simulink library "wtd_library_ver1"  (R2014b)
settings: Solver=ode45  StartTime=0.0  StopTime=10.0  RelTol=1e-3
undefined symbols (not defined in the file or in its folder): clearaugYMatrix, complexPower, dwo, faultaugYMatrix, genTranReactance, invclearaugYMatrix, invfaultaugYMatrix, invsystemaugYMatrix, j, nodeVoltage, noGridNodes, pffault_set_global, s3cc, tho
undefined symbols (not defined in the file): baseSystemPower, internalGenVoltage, pitchAngleVec, systemFrequency, turbSpeedVec, windturbKaParam, windturbKbParam, WTD_Y12, WTD_Y12_2
libraries: simulink x18
(part 1 of 3)
settings Model: Creator=Jakub  LastModifiedBy=Jakub

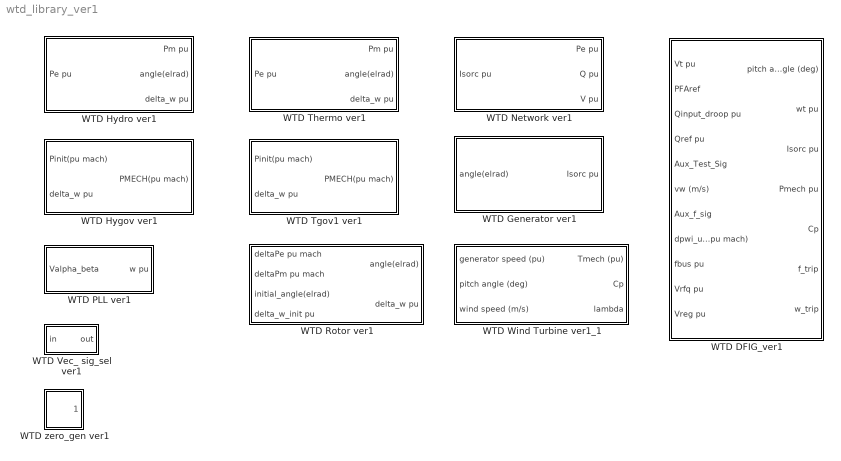
== system wtd_library_ver1 ==
  WTD DFIG_ver1 : Subsystem  mask{co_node=4, Sbasesys=baseSystemPower, Sbasem4=100.5, wbase=2*pi*systemFrequency, H=4.94, Xsecsys=genTranReactance, Ka=windturbKaParam, Kb=windturbKbParam, Vwinit=nodeVoltage, Pelec4abs=real(complexPower)*baseSystemPower, Qgen4abs=imag(complexPower)*baseSystemPower, theta=pitchAngleVec, w=turbSpeedVec, pfaflg=0, varflg=1, apcflg=0, Kqd=0, Kpv=18, Kiv=5, Qmax=0.436, Qmin=-0.436, KVi=40, insupp=0, wi_user_GE=0, Kwi=10, Kptrq=3, Kitrq=0.6, Tpc=0.05, dbwi=0.0025, TIpwi=1, Twowi=5.5, urlwi=0.1, drlwi=-1, Pmxwi=0.1, Pmnwi=0}
      mask prompts: co_node "Connection node number"; Sbasesys "Base system power (MVA)"; Sbasem4 "Nominal machine power (MVA)"; wbase "Base system speed"; H "Machine inertial constant H (s)"; Xsecsys "xdprim (pu sys)"; Vwinit "Initial bus voltage (pu real+j*imag)"; Pelec4abs "Initial active power (MW)"; Qgen4abs "Initial reactive power (MVAr)"; theta "Inital pitch angle (rad)"; w "Inital wind turbine speed (pu)"; pfaflg "Power factor regulation or Q regulation (pfaflg)"; varflg "Voltage regulation, PFA or Q, Q sep. mod. (varflg)"; apcflg "Active power control enabled (apcflg)"; Kqd "Q droop gain Kqd"; Kpv "Reactive power control Kpv"; Kiv "Reactive power control Kiv"; Qmax "Reactive power control qmax"; Qmin "Reactive power control qmin"; KVi "Electrical control Kvi"; insupp "Inertial support (yes = 1, no = 0)"; wi_user_GE "Inertial support: Ge - 0 or User - 1"
      mask init:
      | %DFIG state initialization 
      | %%Generator Converter Model GE
      |     Tcon=0.02;     %converter time constant (s)
      |     %LVPL (low voltage power logic)
      |     zerox=0.2; %0.5  
      |     brkpt=0.9;
      |     LVPLhigh=1.22;
      |     LVPLlow=0;
      |     rrpwr=10;
      |     %Low voltage active current management
      |     lvpnt0=0;%0.4 %Low voltage active current management breakpoint (pu)
      |     lvpnt1=0.8; %Low voltage active current management breakpoint (pu)
      |     klvacm=1/(lvpnt1-lvpnt0);
      |     nlvacm=-lvpnt0/(lvpnt1-lvpnt0);
      |     %High voltage reactive current management
      |     khv=0.7;   %High voltage clamp logic acceleration factor
      |     volim=1.2; %Voltage limit forh high clamp logic (pu on mbase)
      |     iolim=1.5; %Current limit for high voltage clamp logic (pu on mbase)
      |                % -1.0 to -1.5
      | %%Converter Control Model GE
      |     %WindCONTROL Emulator
      |     Tr=0.02; %(s)
      |     Tv=0.05; %(s)
      |     fn=1;
      |     Tc=0.15; %(s)
      |     %Kpv=18; %25
      |     %Kiv=5;
      |     %Qmax=0.436;  %0.52;%(pu),with wind free control 0.12 pu
      |     %Qmin=-0.436; %-0.39;%(pu),with wind free control -0,12.pu
      |     Xc=0;        %(pu)
      |     Vermn=-0.1;  %(pu)
      |     Vermx=0.1;   %(pu)
      |     Vfrz=0.7;    %(pu)
      |     %Power Factor Regulator
      |     Tpwr=0.05;   %(s)
      |     %Q Droop Function Model
      |     TIpqd=5;     %(s)
      |     %Kqd=0;       %0.04;% Q droop off
      |     Xqd=0;
      |  %%Electrical Control
      |     if pfaflg==0 && varflg==0       %Active power regulation
      |         KQi=0.001;    %0.1 or 0.5 for Europen 
      |         %disp('Active power regulation')
      |     elseif pfaflg==0 && varflg==1   %Voltage regulation
      |         KQi=0.1;     %0.001 for North American or 0.5 for Europen
      |         %disp('Voltage regulation')
      |     elseif pfaflg==1 && varflg==0   %Regulation of cosfi
      |         KQi=0.001;    %0.1ili 0.5 for Europen 
      |         %disp('Regulation of cos(fi)')
      |     end
      |     %KVi=40;       %40
      |     KPiadd=0; %8   %Additional P controler for calculation Eqcmd, in generic KVp
      |     XIQmax=+1.45;  %
      |     XIQmin= -0.5;  %0.5
      |     Vmax=1.1;
      |     Vmin=0.9;
      |     IPmax=1.22;
      |     %%Wind Turbine and Turbine control model
      |     %Wind Inertia Control (optional)
      |     %dbwi=0.0025;         % 0.0025 according to lit; 
      |     %TIpwi=1;             % 1 according to lit
      |     %Twowi=5.5;%1.13;     % 5.5 according to lit
      |     %urlwi=0.1;%0.03;     % 0.1 according to lit
      |     %drlwi=-1;%-0.013;    % -1 according to lit
      |     %Pmxwi=0.1;
      |     %Pmnwi=0;
      | %%%%%%%%%%%%%%%%%%%%%%%%%%%%%%%%%%%%%%%%%%%%%%%%%%%%%%%%%%%%%%%%%%%%%%%%
      | %%%%%%%%%%%%%%%%% Wind turbine control parameters%%%%%%%%%%%%%%%%%%%%%%%
      |     %H=5.23;    %Inertial constant for DFIG 3.6MW 60 Hz (H=5.74 for 50Hz)
      |     wrefgr=1.2; %Reference turbine speed, at active power Pelec = 0.457.     
      |     Kpp=150;
      |     Kip=25;
      |     Tp=0.3;
      |     thetamax=27;
      |     thetamin=0;
      |     dtheta_dtmax=10;
      |     dtheta_dtmin=-dtheta_dtmax;
      |     Pwmax=1.12;
      |     Pwmin=0.04;
      |     dP_dtmax=0.45;
      |     dP_dtmin=-0.45;
      |     Kpc=3;
      |     Kic=30;
      |     Prated=1;
      |     donjilimitB=-inf;    %Lower limit of integrator in pitch compensation
      |     upltpitchcont=+inf;  %Upper limit of saturation of pitch controler
      |     lowltpitchcont=-inf; %Lower limit of saturation of pitch controler
      |     upltpitchcomp=+inf;  %Upper limit of saturation of pitch compensation
      |     lowltpitchcomp=-inf; %Lower limit of saturation of pitch compensation
      | %Wind model coefficients
      |     alpha=[-4.1909*10^(-1),2.1808*10^(-1),-1.2406*10^(-2),-1.3365*10^(-4),1.1524*10^(-5);
      |            -6.7606*10^(-2),6.0405*10^(-2),-1.3934*10^(-2),1.0683*10^(-3),-2.3895*10^(-5);
      |            1.5727*10^(-2),-1.0996*10^(-2),2.1495*10^(-3),-1.4855*10^(-4),2.7937*10^(-6); 
      |            -8.6018*10^(-4),5.7051*10^(-4),-1.0479*10^(-4),5.9924*10^(-6),-8.9194*10^(-8); 
      |            1.4787*10^(-5),-9.4839*10^(-6),1.6167*10^(-6),-7.1535*10^(-8),4.9686*10^(-10)];
      | %%Active Power Control (optional)
      |     Tw=1;
      |     Tpav=0.15;
      |     Pa=1;
      |     Pbc=0.95;
      |     Pd=0.4;
      |     Fa=0.96;
      |     Fb=0.996;
      |     Fc=1.004;
      |     Fd=1.04;
      |     Pmax=1;
      |     Pmin=0.2;
      | %GE inertial support
      |     %if insupp == 1   % Ge inertial support is active
      |         % Kwi=35; 
      |         % Kptrq=0.5;  
      |         % Kitrq=0.05;
      |         % Tpc=4; 
      |     %elseif insupp==0 
      |         %Kwi=0;
      |         %Kptrq=3        %Wind inertia control is not active
      |         %Kitrq=0.6      %Wind inertia control is not active
      |         %Tpc=0.05       %Wind inertia control is not active
      |     %end
      | 
      | %% DFIG state initialization
      |                 Pdbr=0;                            %pu mach
      |                 Qgen4=Qgen4abs(co_node)/Sbasem4;   %Initial reactive power
      |                 %pu mach
      |                 Pelec4=Pelec4abs(co_node)/Sbasem4; %Initial active power
      |                 % pu mach
      |                 Xsec=abs(Xsecsys(co_node))*Sbasem4/Sbasesys; %Wind generator equivalent reactance pu machine base
      |                 V4=abs(Vwinit(co_node));           %Voltage at WTG bus
      |                 Vterm4=V4;
      |                 %Wind turbine
      |                 Pmech4=Pelec4+Pdbr;                %Initial mechanical power pu mach
      |                 s0wt=theta(co_node);               %Initial pitch angle
      |                 s6wt=w(co_node);                   %Initial turbine speed
      |                 %Generator/converter model
      |                 %disp('Complex power after shunt reactance Xsec')
      |                 Sgen4=Pelec4+1i*Qgen4;
      |                 %disp('Reactive power into shunt reactance Xsec')
      |                 Sx4=(abs(Vwinit(co_node)))^2/(-1i*Xsec);
      |                 %disp('Complex power in front of shunt reactance Xsec')
      |                 Selec4=Sgen4+Sx4;
      |                 %disp('Power factor cos(fi)')
      |                 %cosfi=Pelec4/abs(Sgen4);
      |                 s0gc=Xsec*imag(Selec4)/Vterm4;
      |                 s1gc=real(Selec4)/Vterm4;
      |                 s2gc=Vterm4;
      |                 %Converter control model
      |                 s1cc=s0gc;                %Eqcmd
      |                 s0cc=Vterm4;              %Vref
      |                 Pord=s1gc*Vterm4; %=Pelec4 in the case that Vterm4=V(4)=real number.
      |                 Qord=Qgen4;
      |                 s6cc=Pelec4;
      |                 s7cc=0; %Q droop
      |                 s5cc=Qord;
      |                 s2cc=0;
      |                 s4cc=s5cc-s2cc;
      |                 %s3cc=Vreg4;
      |                  %Wind inertia control
      |                  s13wt=0;
      |                  s12wt=0;
      |                  pinp=Pord;
      |                  s4wt=pinp;
      |                  s2wt=s4wt/w(co_node);
      |                  %Active power control
      |                  pstl=Prated;
      |                  s11wt=Pmech4;        
      |                  %Wind turbine 
      |                      %Power response rate limiter
      |                      s10wt=0;
      |                      %Pitch compensation and pitch controller
      |                      if (pinp-pstl) < 0
      |                        s3wt=-Kpc*(pinp-pstl); %Initial values of pitch compensator
      |                        s1wt=0;                %Inital value of pitch controller
      |                      else
      |                         s3wt=theta(co_node);
      |                         s1wt=0;
      |                      end
      |                  wref=w(co_node);
      |                  s5wt=wref;
      mask Help:
      | DFIG (according to WTD Library Tutorial Ref. 1)
      | 
      | 
      | PARAMETERS, REGULATION CHOICES, INERTIAL SUPPORT (see Ref. 1)
      | 
      | INPUTS:
      | Vt pu : Complex voltage (pu) of DFIG terminal node
      | PFAref : Reference power factor
      | Qref : Reference reactive power (pu)
      | Aux_Test_sig : See Ref. 1 (usually zero)
      | vw (m/s) : Wind speed (m/s)
      | Aux_f_sig : See Ref. 1 (usually zero)
      | pwi_user (pu mach) : User additional power reference for inertial support (pu mach)
      | fbus pu : DFIG connection node voltage frequency pu of system base frequency
      | Vrfq pu : Reference of complex voltage which is controlled
      | Vreg pu : Measured complex voltage which is controlled
      | 
      | OUTPUTS:
      | pitch angle (deg) : Pitch angle deg
      | wt pu : Turbine speed pu
      | Isorc pu : Current of DFIG current source pu
      | Pmech pu : Turbine mechanical power pu
      | Cp : Power factor
      | f_trip : Frequency trip signal ( = 1 if network frequency is higher than 1.04 pu for more than 1 sec, otherwise = 0)
      | w_trip : Turbine speed trip signal ( = 1 if turbine speed is less than 0.2 pu)
      | 
      | NOTES:
      | WTG initial speed, WTG initial pitch angle, initial wind speed, initial active and
      | reactive power are initialized by the Network block.
      | LVRT and HVRT capabilities are not supported. These capabilities can be programmed externally.
      | Pseudo Drag Term is not realized.
      | WindFree operation is not supported.
      | Open Loop Reactive Power Control is not supported.
      | Power flow and initial conditions are calculated, using Network block, with assumption that
      | Active Power Control (APC) is disabled (apcflg = 0), regardless of the APC is enabled (apcflg = 1) or disabled.
      | If APC is enabled then in the first moments of a simulation there is transition process to the steady state.
      | In order to use Wind Inertia (WI), parameter Kwi must be set to value > 0 and parameter Inertial support must be set to 1.
      | There are two possibilities for Inertial support: General Electric algorithm generated inertial support signal or
      | User inertial support algorithm generated inertial support signal. In order to use User inertial support generated signal,
      | this signal must be connected to the input dpwi_user (pu mach) of DFIG block. In the case of using GE inertial support,
      | default values of the parameters are: Kptrq = 3, Kitrq = 0.6 and Tpc =0.05 should be changed to the values:
      | Kptrq = 0.5;
      | Kitrq = 0.05;
      | Tpc = 4;
  WTD Generator ver1 : Subsystem  mask{co_node=1, E=internalGenVoltage, jxd=genTranReactance}
      mask prompts: co_node "Connection node number"; E "E pu sys"; jxd "jXd pu sys"
      mask init:
      | abs_Eprim=abs(E(co_node));
      mask Help:
      | Generator block
      | 
      | 
      | Generator block includes E' behind Xd' generator model.
      | 
      | PARAMETERS:
      | Conection node number: Number of the node of network where generator is connected
      | E pu: Transient voltage of generator pu (disabled)
      | jXd pu: Generator transient reactance pu (disabled)
      | 
      | INPUTS:
      | angle(elrad): Rotor/generator angle in electrical radians
      | 
      | OUTPUTS:
      | Isorc pu: Current of an equivalent current generator
      | 
      | NOTES:
      | Generator block is initialized by the Network block.
  WTD Hydro ver1 : Subsystem  mask{co_node=1, Sbasesys=baseSystemPower, Sbasem1=247.5, wbase=2*pi*systemFrequency, H1=2364/247.5, D1=2, Pm_init_vec=real(complexPower)*baseSystemPower, delta_init_vec=angle(internalGenVoltage), R11=0.05, r1=0.4, Tr1=8, Tf1=0.05, Tg1=0.2, VELM1=0.2, Gmax1=1, Gmin1=0, Tw1=1.2, Dturb1=0, At1=1, qNL1=0.068}
      mask prompts: co_node "Connection node number"; Sbasesys "Base system power  (MVA)"; Sbasem1 "Nominal machine power (MVA)"; wbase "Base system speed (rad/s)"; H1 "Machine inertial constant H (s)"; D1 "Load/Machine damping D pu"; Pm_init_vec "Initial mechanical power vector(MW)"; delta_init_vec "Initial rotor angle vector (rad)"; R11 "Permanent droop (R)"; r1 "Temporary droop (r)"; Tr1 "Governor time constant (Tr)"; Tf1 "Filter time constant (Tf)"; Tg1 "Servo time constant (Tg)"; VELM1 "Gate velocity limit (VELM)"; Gmax1 "Maximum gate limit (Gmax)"; Gmin1 "Minimum gate limit (Gmin)"; Tw1 "Water time constant (Tw)"; Dturb1 "Turbine damping (Dturb)"; At1 "Turbine gain (At)"; qNL1 "No power flow (qNL)"
      mask Help:
      | Hydro block
      | 
      | 
      | Hydro turbine/governor/rotor model
      | 
      | Model includes HYGOV PSS model, and rotor/load damping (D) model.
      | 
      | For explanation of the parameters of the block see PSS/E documentation (Ref. 2).
  WTD Hygov ver1 : Subsystem  mask{R11=0.05, r1=0.4, Tr1=8, Tf1=0.3125, Tg1=0.2, VELM1=0.5, Gmax1=2, Gmin1=0, Tw1=1.2, Dturb1=0, At1=2.5, qNL1=0.068}
      mask prompts: R11 "Permanent droop (R)"; r1 "Temporary droop (r)"; Tr1 "Governor time constant (Tr)"; Tf1 "Filter time constant (Tf)"; Tg1 "Servo time constant (Tg)"; VELM1 "Gate velocitiy limit (VELM)"; Gmax1 "Maximum gate limit (Gmax)"; Gmin1 "Minimum gate limit (Gmin)"; Tw1 "Water time constant (Tw)"; Dturb1 "Turbine damping (Dturb)"; At1 "Turbine Gain (At)"; qNL1 "No power flow (qNL)"
      mask Help:
      | Hygov Block
      | 
      | 
      | Model includes HYGOV PSS turbine-governor model
      | For explanation of the parameters see PSS/E documentation (WTD Library Tutorial Ref. 2)
  WTD Network ver1 : Subsystem  mask{Sbasesys=100, fsystem=50, Ydf=WTD_Y12, no_gen_co=3, no_gen_wi=1, nodes_co=[2,1,3], xd_co=[0.1198,0.0608,0.1813], nodes_wi=4, Pbasemw=100, xd_wi=0.8, Ka=0.00159, Kb=56.6, nodes_lo=[6,5,8], Sloadabs=[90+j*30,125+j*50,100+j*35], flttype=Power, Tfault=3, nodeadd=8, Saddabs=10, fltimp=10.32, linenumber=1, Tclear=inf, Y2df=WTD_Y12_2, absV_co=[1.025,1.04,1.025], Sgenabs_co=[103,0,85], wi_choice=Active_power, absV_wi=1.031, Sgenabs_wi=60, vw_vector=14, pfcalc=off, pffault=on}
      mask prompts: Sbasesys "Base system power (MVA)"; fsystem "System frequency (Hz)"; Ydf "Name  of the network description csv file"; no_gen_co "Number of conventional generators"; no_gen_wi "Number of wind generators"; nodes_co "Conventional generators nodes row vector"; xd_co "Conventional generators transient reactance row vector Xd pu sys"; nodes_wi "Wind generators nodes row vector"; Pbasemw "Wind generators nominal power row vector (MVA)"; xd_wi "Wind generators shunt reactance row vector Xd pu sys"; Ka "Wind generators Ka constant row vector"; Kb "Wind generators Kb constant row vector"; nodes_lo "Load nodes row vector"; Sloadabs "Complex power load row vector (MVA)"; flttype "Type of the fault"; Tfault "Fault time"; nodeadd "Faulted node number"; Saddabs "Fault node additional power (MVA)"; fltimp "Fault node impedance pu sys"; linenumber "Disconnect line identification number"; Tclear "Clear time"; Y2df "Name of the network post clear fault description csv file"; absV_co "Conventional generator nodes initial voltages row vector pu"; Sgenabs_co "Conventional generator nodes initial active power row vector (MW)"; wi_choice "Wind generator initial conditions"; absV_wi "Wind generator nodes initial voltages row vector pu"; Sgenabs_wi "Wind generator nodes initial active power row vector (MW)"; vw_vector "Wind generator initial wind speed row vector (3m/s<v<25m/s)"; pfcalc "Initialization and power flow calculation"; pffault "Additional iterations at the start and at the end of the fault ?"
      mask init:
      | no_generators=no_gen_co+no_gen_wi;
      mask Help:
      | Network block
      | Author: Jakub Osmic
      | 
      | Network block enables input of data required to perform power flow calculation.
      | Apart from this, data on disturbances, short circuit and reconfiguration of the network
      | (disconnection of a transmission line) can be entered.
      | This block solves the network voltage equations during a simulation.
      | In addition, this block calculates initial data for turbines, conventional generators and wind generators.
      | For any simulation of the dynamic response of WTG, the Network block must be included.
      | Before simulation is started, it is necessary to perform power flow calculation using the Network block.
      | 
      | NOTES:
      | The generator nodes must be in the order of 1 and further.
      | The slack node must be the node number 1.
      | At minimum one generator must be connected to the network.
      | Precisely one generator is a slack generator (with an internal voltage angle equal to 0 rad).
      | All input and output signals are pu of the system base quantities.
      | 
      | PARAMETERS:
      | The network model accepts parameters either as variable names or as variable values that can be scalars or vectors.
      | 
      | INPUTS:
      | Isorc pu: Multiplexed input of complex currents of the equivalent current generators.
      | The inputs must be multiplexed so that input of the first generator is connected to the first node and so on.
      | In each node of Network block, current source can be connected. If no current source is connected to appropriate node,
      | ZERO_GEN block must be connected. The overall number of Generator blocks and ZERO_GEN blocks must be equal to the number of network nodes.
      | 
      | OUTPUTS:
      | Pe pu: Output vector of active power injected into the nodes of the network.
      | To select power injected to any node, this output must be connected to the input of Vec. Sig. Selector block located in the WTD Library.
      | As a parameter of this block, select the order number of the node in which the specified power is to be injected.
      | Qe pu: Similar to the previous one. Qe represents the vector of the reactive power injected into the nodes of the network.
      | V pu: Similar to the previous one. V represents complex vector of node voltages.
      | 
      | Network tab
      | Name of network description file: A name of the csv file (without quotation and without extension) by which the network is described.
      | This block accepts a name of network description file so that the first character must be a letter (excluding special characters and space character).
      | The file is created by a text editor by putting csv file extension, or by using MS EXCEL. The sheet name is the same as the name of the file.
      | The file contents is as follows:
      | 
      | line order number, sending node order number, receiving node order number, line impedance (pu) (eg. 0.1+j*0.1 or 0.1+i*0.1), line susceptance j*B/2 (pu), shunt admittance (pu) both in the sending and receiving nodes
      | ...
      | line order number, sending node order number, receiving node order number, line impedance (pu) (eg. 0.1+j*0.1 or 0.1+i*0.1), line susceptance j*B/2 (pu), shunt admittance (pu) both in the sending and receiving nodes
      | 
      | Line susceptance and shunt admittance in a j-th row of the network description file adds up to i-th diagonal element of network admittance matrix every time when there is number i (i-th node order number) in the second or the third column of the j-th row of the network description file.
      | The file must be saved in the Working directory. Based on this file,
      | the Network block calculates the matrix of the network admittances.
      | 
      | Number of conventional generators: Enter the number of conventional generators (minimum 1).
      | 
      | Number of wind generators: Enter the number of wind generators, 0 if there is no wind generators.
      | 
      | Generators Conv. tab
      | Conventional generators nodes row vector: Enter nodes of conventional generators in square brackets with space or comma
      | (eg. [2 1 3] or [2,1,3]). If there is one generator then the number of node can be entered without brackets.
      | Conventional generators transient reactance row vector Xd pu sys:
      | Enter the row vector of transient reactance of conventional generators
      | in the same order as the order of generator connection nodes.
      | 
      | Wind Gener. tab
      | Wind generators nodes row vector: See GENERATORS CONV.
      | Wind generators nominal power row vector (MVA): Enter the row vector of the nominal power of the wind generators.
      | Wind generators shunt reactance row vector Xd pu sys: See GENERATORS CONV.
      | Wind generators Ka constant row vector: Enter vector of Ka constants of wind generators (see Ref. 1). Ka=1/2*rho*A.
      | Wind generators Kb a constant row vector: Enter vector of Kb constants of wind generators (see Ref. 1). lambda = Kb*omega(pu)/wind speed (m/s).
      | 
      | Load tab
      | Load nodes row vector: Enter row vector of nodes in which loads are connected. The vector is entered as in the previous cases.
      | If there are no nodes with loads then place the empty brackets [].
      | Complex power load vector (MVA): Enter row vector of complex load power in MVA (eg 50 + j * 35) in the same order as input load nodes.
      | If there are no load nodes enter empty brackets [].
      | A load cannot be added to the generator node.
      | 
      | Fault tab
      | Type of the fault: Power, Short circuit or Line disconnection. This menu allows to select the three types of disturbances / faults.
      | In the case of selecting Power fault/distrubance, a complex disturbance power may be entered in the MVA (eg 10 + j * 5).
      | In a case of selecting Short circuit it is possible to enter fault impedance (pu sys). Take care that the fault impedance is higher than zero!
      | Fault time: Enter the time when a disturbance occurs. Enter inf if there is no fault (fault is in infinity).
      | Faulted node number: Enter number of a node in which the fault appears (the node number input is obligatory).
      | Fault node additional power: Enter the complex power of disturbance in the MVA. On the basis of this power,
      | impedance of the fault is calculated using the node voltage before the fault. This entry is mandatory.
      | Disconnect line identification number: Enter the line number of the line that is disconnected (only one line can be disconnected at the time).
      | Clear time: Enter the time when the fault is cleared. In the case that the fault will last forever, enter inf (mandatory input).
      | Csv file: See the NETWORK: Name of the network description file
      | 
      | Power Flow tab
      | Conventional generator nodes initial voltages row vector pu sys: The modules of voltages of the PV nodes are accepted
      | in the same format and in the same order as the connecting nodes of conventional generators (see Generators conv.)
      | Conventional generator nodes initial active power row vector (MW): Initial active power of conventional generators in MW
      | in the same order and in the same format as the connecting nodes of conventional generators.
      | Wind generator initial conditions: Two choices are possible: Active power or Wind speed.
      | In the case of the first choice, it is possible to input the initial active wind turbine power in MW.
      | In case of a second choice, it is possible to input the initial wind speed.
      | Wind generators nodes initial voltages row vector pu: The modules of voltages of the PV nodes where wind generators are connected pu sys.
      | 
      | Initialization and Power Flow Calculation: By selecting this field, the power flow calculations and initialization of the wind
      | turbine/generator speed, pitch angle and initial wind speed (or initial active power) are performed.
      | All required variables are recorded in the Workspace (the meaning of the variable is clear from their names):
      | baseSystemPower: System base power in MVA
      | clearaugYMatrix: Network admittance matrix with included generator and load admittances after clearance of the fault
      | clearfaultYMatrix: Network admittance matrix after clearance of the fault
      | complexPower: Vector of complex powers injected into the nodes
      | faultaugYMatrix: Network admittance matrix with included generator and load admittances after the fault
      | genTranReactance: Vector of generator transient reactance xd'
      | internalGenVoltage: Vector of E' of generator internal voltages
      | invclearaugYMatrix: Inversion of clearaugYMatrix matrix
      | invfaultaugYMatrix: Inversion of faultaugYMatrix
      | invsystemaugYMatrix: Inversion of systemaugYMatrix
      | noGridNodes: Number of grid nodes
      | nodeVoltage: Vector of phasors of node voltages
      | pitchAngleVec: Vector of initial pitch angles of wind turbines
      | systemFrequency: System frequency
      | systemYMatrix: Network admittance matrix (before the fault)
      | systemaugYMatrix: Network admittance matrix with included generator and load admittances (before fault)
      | turbSpeedVec: Vector of initial speed of wind turbine/generators
      | windSpeedVec: Vector of initial wind speed of wind turbine/generators
      | windturbKaParam: Vector of Wind turbines Ka parameters (see Ref. 1)
      | windturbKbParam: Vector of Wind turbines Kb parameters (Ref. 1)
      | 
      | In order to re-execute the power flow calculations, the field must first be deselected and re-selected.
      | The rule is: after any changes to entries in Network block it is necessary to re-initialize and re-calculate
      | power flow by selecting the appropriate field. By closing the Network block dialog box, this field is automatically deselected.
      | In each iteration node voltages are calculated by using formula
      | nodeVoltage=invsystemaugYMatrix*Isorc
      | Where invsystemaugYMatrix is inversion of the network admittance matrix with included load admittances and generator admittances.
      | 
      | Additional iterations at the start and at the end of fault?:
      | By selecting this field additional iterations (during the two Simulink steps) are performed by using Gauss Siedel
      | algorithm with constraints. In the most of the cases this functionality can reduce peaks in the voltage and electrical power response,
      | immediately after fault or immediately after the fault clearance.
      | The peaks are result of the fact that in the iterations of network equations the equations of Low Voltage Active Current Management
      | and High Voltage Reactive Current Management are not included(they are included in the WTG model).
      mask Callback Sbasesys:
      | set_param(gcb,'pfcalc','off')
      | %set_param(gcb,'pffault','off')
      mask Callback no_gen_co:
      | if ~isempty(str2num(get_param(gcb,'no_gen_co')))
      | maskVi=get_param(gcb,'MaskVisibilities');
      | if str2num(get_param(gcb,'no_gen_co'))==0
      | maskVi{6}='off';
      | maskVi{7}='off';
      | maskVi{23}='off';
      | maskVi{24}='off';
      | set_param(gcb,'MaskVisibilities',maskVi)
      | elseif (str2num(get_param(gcb,'no_gen_co'))==1)...
      |         && isempty(str2num(get_param(gcb,'no_gen_wi')))
      | maskVi{6}='on';
      | maskVi{7}='on';
      | maskVi{23}='on';
      | maskVi{24}='off';
      | set_param(gcb,'MaskVisibilities',maskVi)
      | elseif (str2num(get_param(gcb,'no_gen_co'))==1)...
      |             && (str2num(get_param(gcb,'no_gen_wi'))==0)
      | maskVi{6}='on';
      | maskVi{7}='on';
      | maskVi{23}='on';
      | maskVi{24}='off';
      | set_param(gcb,'MaskVisibilities',maskVi)
      | else
      | maskVi{6}='on';
      | maskVi{7}='on';
      | maskVi{23}='on';
      | maskVi{24}='on';
      | set_param(gcb,'MaskVisibilities',maskVi)
      | end
      | clear maskVi
      | end
      mask Callback no_gen_wi:
      | if ~isempty(str2num(get_param(gcb,'no_gen_wi')))
      | maskVi=get_param(gcb,'MaskVisibilities');
      | if str2num(get_param(gcb,'no_gen_wi'))==0
      | maskVi{8}='off';
      | maskVi{9}='off';
      | maskVi{10}='off';
      | maskVi{11}='off';
      | maskVi{12}='off';
      | maskVi{25}='off';
      | maskVi{26}='off';
      | maskVi{27}='off';
      | maskVi{28}='off';
      | set_param(gcb,'MaskVisibilities',maskVi)
      | else
      | maskVi{8}='on';
      | maskVi{9}='on';
      | maskVi{10}='on';
      | maskVi{11}='on';
      | maskVi{12}='on';
      | maskVi{25}='on';
      | maskVi{26}='on';
      | maskVi{27}='on';
      | maskVi{28}='on';
      | set_param(gcb,'MaskVisibilities',maskVi)
      | end
      | clear maskVi
      | end
      mask Callback nodes_co:
      | if ~isempty(str2num(get_param(gcb,'nodes_co')))
      | maskVi=get_param(gcb,'MaskVisibilities');
      | if (str2num(get_param(gcb,'no_gen_co'))==1)...
      |         && (str2num(get_param(gcb,'nodes_co'))==1)
      | maskVi{24}='off';
      | set_param(gcb,'MaskVisibilities',maskVi)
      | else
      | maskVi{24}='on';
      | set_param(gcb,'MaskVisibilities',maskVi)
      | end
      | clear maskVi
      | end
      mask Callback nodes_wi:
      | if ~isempty(str2num(get_param(gcb,'nodes_wi')))
      | maskStr=get_param(gcb,'MaskValues');
      | maskVi=get_param(gcb,'MaskVisibilities');
      | if str2num(get_param(gcb,'no_gen_wi'))==0
      | maskVi{8}='off';
      | maskVi{9}='off';
      | maskVi{10}='off';
      | maskVi{11}='off';
      | maskVi{12}='off';
      | maskVi{25}='off';
      | maskVi{26}='off';
      | maskVi{27}='off';
      | maskVi{28}='off';
      | set_param(gcb,'MaskVisibilities',maskVi)
      | elseif any(str2num(get_param(gcb,'nodes_wi'))==1)
      | maskVi{8}='on';
      | maskVi{9}='on';
      | maskVi{10}='on';
      | maskVi{11}='on';
      | maskVi{12}='on';
      | set_param(gcb,'wi_choice','Active_power')
      | maskVi{25}='off';
      | maskVi{26}='on';
      | maskVi{27}='on';
      | maskVi{28}='off';
      | set_param(gcb,'MaskVisibilities',maskVi)
      | elseif  strcmp(maskStr{25}(1),'A')
      | maskVi{8}='on';
      | maskVi{9}='on';
      | maskVi{10}='on';
      | maskVi{11}='on';
      | maskVi{12}='on';
      | maskVi{25}='on';
      | maskVi{26}='on';
      | maskVi{27}='on';
      | maskVi{28}='off';
      | set_param(gcb,'MaskVisibilities',maskVi)
      | elseif  strcmp(maskStr{25}(1),'W')
      | maskVi{8}='on';
      | maskVi{9}='on';
      | maskVi{10}='on';
      | maskVi{11}='on';
      | maskVi{12}='on';
      | maskVi{25}='on';
      | maskVi{26}='on';
      | maskVi{27}='off';
      | maskVi{28}='on';
      | set_param(gcb,'MaskVisibilities',maskVi)
      | end
      | clear maskVi maskStr
      | end
      mask TypeOptions flttype: Power | Short_circuit | Line_disconnect
      mask Callback flttype:
      | maskStr=get_param(gcb,'MaskValues');
      | maskVi=get_param(gcb,'MaskVisibilities');
      | if strcmp(maskStr{15}(1),'P')
      | maskVi{17}='on';
      | maskVi{18}='on';
      | maskVi{19}='off';
      | maskVi{20}='off';
      | set_param(gcb,'MaskVisibilities',maskVi)
      | elseif strcmp(maskStr{15}(1),'S')
      | maskVi{17}='on';
      | maskVi{18}='off';
      | maskVi{19}='on';
      | maskVi{20}='off';
      | set_param(gcb,'MaskVisibilities',maskVi)
      | elseif strcmp(maskStr{15}(1),'L')
      | maskVi{17}='off';
      | maskVi{18}='off';
      | maskVi{19}='off';
      | maskVi{20}='on';
      | set_param(gcb,'MaskVisibilities',maskVi)
      | end
      | clear maskVi maskStr
      mask TypeOptions wi_choice: Active_power | Wind_speed
      mask Callback wi_choice:
      | maskStr=get_param(gcb,'MaskValues');
      | maskVi=get_param(gcb,'MaskVisibilities');
      | if ~isempty(str2num(get_param(gcb,'no_gen_wi')))
      |     if str2num(get_param(gcb,'no_gen_wi'))==0
      |     maskVi{25}='off';
      |     maskVi{26}='off';
      |     maskVi{27}='off';
      |     maskVi{28}='off';
      |     elseif strcmp(maskStr{25}(1),'A')
      |     maskVi{25}='on';
      |     maskVi{26}='on';
      |     maskVi{27}='on';
      |     maskVi{28}='off';
      |     set_param(gcb,'MaskVisibilities',maskVi)
      |     elseif strcmp(maskStr{25}(1),'W')
      |     maskVi{25}='on';
      |     maskVi{26}='on';
      |     maskVi{27}='off';
      |     maskVi{28}='on';
      |     set_param(gcb,'MaskVisibilities',maskVi)
      |     end
      | elseif isempty(str2num(get_param(gcb,'no_gen_wi'))) && ...
      |     strcmp(maskStr{25}(1),'A')
      |     maskVi{25}='on';
      |     maskVi{26}='on';
      |     maskVi{27}='on';
      |     maskVi{28}='off';
      |     set_param(gcb,'MaskVisibilities',maskVi)
      | elseif isempty(str2num(get_param(gcb,'no_gen_wi'))) &&...
      |     strcmp(maskStr{25}(1),'W')
      |     maskVi{25}='on';
      |     maskVi{26}='on';
      |     maskVi{27}='off';
      |     maskVi{28}='on';
      |     set_param(gcb,'MaskVisibilities',maskVi)
      | end
      | clear maskVi maskStr
      mask Callback pfcalc:
      | if strcmp(get_param(gcb,'pfcalc'),'on')
      | [complexPower,nodeVoltage,internalGenVoltage,...
      |     genTranReactance,systemaugYMatrix,faultaugYMatrix,...
      |     clearaugYMatrix,windSpeedVec,turbSpeedVec,...
      |     pitchAngleVec,noGridNodes,windturbKaParam,...
      |     windturbKbParam,baseSystemPower,systemFrequency,...
      |     systemYMatrix,clearfaultYMatrix,invsystemaugYMatrix,...
      |     invfaultaugYMatrix,invclearaugYMatrix]...
      |  =initGridFunPro_Ver3(@powerFlowFun,@initvwFun,@initPelecFun ,...
      |  @augYFun,@admMatCalcCsv_Ver2);
      |     if ~strcmp(get_param(gcb,'Ydf'),'')
      |     evalc(strcat(get_param(gcb,'Ydf'),'=systemYMatrix'));
      |     end
      |     if ~strcmp(get_param(gcb,'Y2df'),'')
      |     evalc(strcat(get_param(gcb,'Y2df'),'=clearfaultYMatrix'));
      |     end
      | end
      mask Callback pffault:
      | if strcmp(get_param(gcb,'pffault'),'on')
      |    %set_param(gcb,'pffault_set','1')
      |    pffault_set_global=1;
      | else
      |     %set_param(gcb,'pffault_set','0')
      |     pffault_set_global=0;
      | end
  WTD PLL ver1 : Subsystem  mask{me_node=8, KpPLL=30, KiPLL=0, delta_init_vec=angle(nodeVoltage ), wbase=2*pi*systemFrequency}
      mask prompts: me_node "Measurement node number"; KpPLL "Proportional gain"; KiPLL "Integral gain"; delta_init_vec "Initial angle (rad)"; wbase "Base system speed (rad/s)"
      mask Help:
      | PLL block
      | 
      | 
      | PLL (Phase Locked Loop) block is used for measurement frequency of a signal.
      | 
      | PARAMETERS:
      | Measurement node number:  Measurement signal node number
      | Proportional gain: Proportional gain of the PI controller (default 30)
      | Integral gain: Integral gain of PI controller (default 0)
      | 
      | INPUTS:
      | Input in this block is node voltage phasor pu.
      | 
      | OUTPUTS:
      | Output of this block is voltage angle frequency pu filtered by low pass fourth order
      | Buttherworth filter with bandwidth frequency of 25 Hz
  WTD Rotor ver1 : Subsystem  mask{wbase=0, H=0, D=0}
      mask prompts: wbase "Base system speed (rad/s)"; H "Machine inertial constant H (s)"; D "Load damping D pu"
      mask Help:
      | Rotor block
      | 
      | 
      | Single mass turbine/generator rotor/damping (D) model.
      | 
      | PARAMETERS:
      | Base system speed (rad/s)
      | Machine inertial constant H (s)
      | Load damping D pu
      | 
      | INPUTS:
      | deltaPe pu mach: Deviation of electrical power (pu) from initial electrical power, pu of turbine/generator rated power
      | deltaPm pu mach: Deviation of turbine mechanical power from initial, pu of turbine/generator rated power
      | initial_angle(elrad): Rotor initial angle in electrical radians
      | delta_w_init pu: Initial deviation of turbine/generator angle speed, pu of base system speed
      | 
      | OUTPUTS:
      | angle(elrad): Deviation of rotor angle from the initial rotor angle in electrical radians
      | delta_w_init pu: Deviation of turbine/generator angle speed from the initial angle speed, pu of the base system speed
  WTD Tgov1 ver1 : Subsystem  mask{R2=0.05, Dt2=0, T12=0.2, T22=0.3*7, T32=7, Vmax2=1, Vmin2=0}
      mask prompts: R2 "Droop R"; Dt2 "Turbine damping Dt"; T12 "T1 (s)"; T22 "T2 (s)"; T32 "T3 (s)"; Vmax2 "Vmax"; Vmin2 "Vmin"
      mask Help:
      | TGOV1 block
      | 
      | 
      | Model includes turbine-governor TGOV1 PSS model
      | 
      | For explanation of the parameters see PSS/E documentation (WTD Library Tutorial Ref. 2)
  WTD Thermo ver1 : Subsystem  mask{co_node=2, Sbasesys=baseSystemPower, Sbasem2=192, wbase=2*pi*systemFrequency, H2=640/192, D2=2, Pm_init_vec=real(complexPower)*baseSystemPower, delta_init_vec=angle(internalGenVoltage), R2=0.05, Dt2=0, T12=0.2, T22=0.3*7, T32=7, Vmax2=1, Vmin2=0}
      mask prompts: co_node "Connection node number"; Sbasesys "Base system power (MVA)"; Sbasem2 "Nominal machine power (MVA)"; wbase "Base system speed (rad/s)"; H2 "Machine inertial constant H (s)"; D2 "Load/Machine damping D pu"; Pm_init_vec "Initial mechanical power (MW)"; delta_init_vec "Initial rotor angle (rad)"; R2 "Droop (R)"; Dt2 "Turbine damping (Dt)"; T12 "T1 (s)"; T22 "T2 (s)"; T32 "T3 (s)"; Vmax2 "Vmax"; Vmin2 "Vmin"
      mask Help:
      | Thermo block.
      | 
      | 
      | Thermo block includes TGOV PSS model and rotor/load damping (D) model.
      | 
      | For explanation of the parameters see PSS/E documentation (Ref. 2)
  WTD Vec_ sig_sel ver1 : Subsystem  mask{node=4}
      mask prompts: node "Node number"
      mask Help:
      | Vec_sig_selector block
      | 
      | 
      | Block selects appropriate node signal from vector node signal input
      | 
      | PARAMETERS:
      | Node number: Number of node which signal belongs to
      | 
      | INPUT:
      | in: Vector signal
      | 
      | OUTPUT:
      | out: Scalar signal output
  WTD Wind Turbine ver1_1 : Subsystem  mask{Pnom=1.5e6, Pelec_base=1.5e6/0.9, wind_base=12, P_wind_base=0.73, speed_nom=1.2, lambda_nom=8.1, cp_nom=0.48}
      mask prompts: Pnom "Nominal mechanical output power (W)"; Pelec_base "Base power of the electrical generator (VA)"; wind_base "Base wind speed v1(m/s)"; P_wind_base "Maximum power at base wind speed (pu of nominal mechanical power)"; speed_nom "Base rotational speed wb(pu of base generator speed)"; lambda_nom "Lambda optimal"; cp_nom "Cp maximum"
      mask init:
      | %Coeficient according to Matlab/Simulink
      | c1=0.51763;
      | c2=116;
      | c3=0.4;
      | c4=5;
      | c5=21;
      | c6=0.006795;
      mask Help:
      | WIND TURBINE block according to Matlab/Simulink documentation
      | 
      | Wind Turbine block is similar to the Simulink/SimPowerSystems/Wind Turbine.mdl block.
      | Wind Turbine block implements the same aerodynamic model used in built in Simulink Wind Turbine.mdl block
      | but has different parameters and outputs.
      | 
      | PARAMETERS :
      | Nominal mechanical output power: The nominal output power in watts (W).
      | Base power of the electrical generator: The nominal power of the electrical generator coupled to the wind turbine, in VA.
      | This parameter is used to compute the output torque in pu of the nominal torque of the generator.
      | Base wind speed v1 (m/s): The base value of the wind speed, in m/s, used in the per unit system.
      | The base wind speed is the mean value of the expected wind speed. This base wind speed produces
      | a mechanical power which is usually lower than the turbine nominal power.
      | Maximum power at base wind speed (pu of nominal turbine power): The maximum power at base wind speed in pu of the nominal mechanical power.
      | Base rotational speed wb (pu of base generator speed): The rotational speed at maximum power for the base wind speed.
      | 
      | For a synchronous or asynchronous generator, the base speed is the synchronous speed.
      | For a permanent-magnet generator, the base speed is defined as the speed producing nominal voltage at  no load.
      | The turbine inertia must be added to the generator inertia.
      | 
      | INPUTS:
      | generator speed (pu): generator speed pu of base generator speed
      | pitch angle (deg): pitch angle in degrees
      | wind speed (m/s): wind speed in m/s
      | 
      | OUTPUTS:
      | Tmech (pu): simulink output of the mechanical torque of the wind turbine, in pu of the nominal generator torque.
      | The nominal torque of the generator is based on the nominal generator power and speed.
      | Cp: power coefficient of turbine (maximum value 0.48 among others @ wind speed = v1, pitch angle = 0 deg and generator speed = wb)
      | lambda : tip speed ratio (optimal value 8.1 among others @ wind speed = v1,
      | generator speed = wb)
  WTD zero_gen ver1 : Subsystem
      mask Help:
      | ZERO_GEN block
      | 
      | 
      | This block represents current source that injects zero current into a
      | network node to which no generator is connected.
      | 
      | It should be connected to Isorc input of the Network block.
      | 
      | The overall number of Generator blocks and ZERO_GEN blocks must be equal to the number of network nodes.
      | 
      | OUTPUT:
      | Isorc : Equal to the complex number 0+j*0

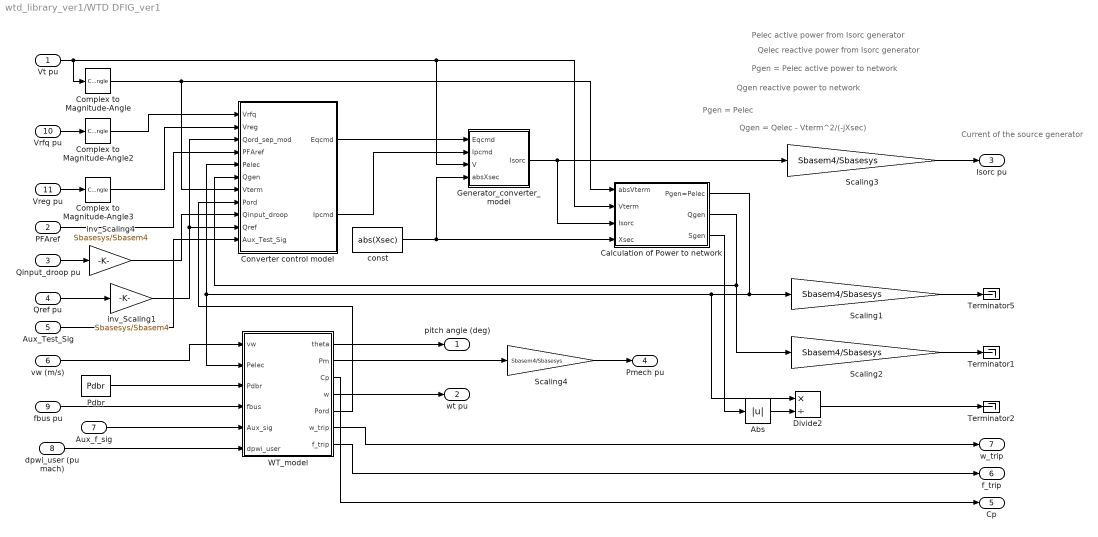
== system wtd_library_ver1/WTD DFIG_ver1 ==
  note: Current of the source generator
  note: Pgen = Pelec
  note: Qgen = Qelec - Vterm^2/(-jXsec)
  note: Pelec active power from Isorc generator
  note: Qelec reactive power from Isorc generator
  note: Pgen = Pelec active power to network
  note: Qgen reactive power to network
  Vt pu : Inport
  PFAref : Inport  Port=2
  Qinput_droop pu : Inport  Port=3
  Qref pu : Inport  Port=4
  Aux_Test_Sig : Inport  Port=5
  vw (m/s) : Inport  Port=6
  Aux_f_sig : Inport  Port=7
  dpwi_user (pu mach) : Inport  Port=8
  fbus pu : Inport  Port=9
  Vrfq pu : Inport  Port=10
  Vreg pu : Inport  Port=11
  Abs : Abs
  "Calculation of Power to network " : Subsystem
  Complex to Magnitude-Angle : ComplexToMagnitudeAngle  Output=Magnitude
  Complex to Magnitude-Angle2 : ComplexToMagnitudeAngle  Output=Magnitude
  Complex to Magnitude-Angle3 : ComplexToMagnitudeAngle  Output=Magnitude
  Converter control model : Subsystem
  Divide2 : Product  Inputs=*/
  Generator_converter_model : Subsystem
  Pdbr : Constant  Value=Pdbr
  Scaling{1..4} (4 alike) : Gain  Gain=Sbasem4/Sbasesys
  Terminator1 : Terminator
  Terminator2 : Terminator
  Terminator5 : Terminator
  WT_model : Subsystem
  const : Constant  Value=abs(Xsec)
  inv_Scaling1 : Gain  Gain=Sbasesys/Sbasem4
  inv_Scaling4 : Gain  Gain=Sbasesys/Sbasem4
  pitch angle (deg) : Outport
  wt pu : Outport  Port=2
  Isorc pu : Outport  Port=3
  Pmech pu : Outport  Port=4
  Cp : Outport  Port=5
  f_trip : Outport  Port=6
  w_trip : Outport  Port=7
  wires:
  Scaling3/1 -> Isorc pu/1
  Scaling4/1 -> Pmech pu/1
  Pdbr/1 -> WT_model/3(Pdbr)
  inv_Scaling1/1 -> Converter control model/10(Qref), Converter control model/3(Qord_sep_mod)
  inv_Scaling4/1 -> Converter control model/9(Qinput_droop)
  const/1 -> Generator_converter_model/4(absXsec), "Calculation of Power to network "/4(Xsec)
  dpwi_user (pu mach)/1 -> WT_model/6(dpwi_user)
  Complex to Magnitude-Angle3/1 -> Converter control model/2(Vreg)
  Vreg pu/1 -> Complex to Magnitude-Angle3/1
  Complex to Magnitude-Angle2/1 -> Converter control model/1(Vrfq)
  Vrfq pu/1 -> Complex to Magnitude-Angle2/1
  Divide2/1 -> Terminator2/1
  Abs/1 -> Divide2/2
  Aux_f_sig/1 -> WT_model/5(Aux_sig)
  fbus pu/1 -> WT_model/4(fbus)
  WT_model/4(w) -> wt pu/1
  WT_model/1(theta) -> pitch angle (deg)/1
  vw (m/s)/1 -> WT_model/1(vw)
  Aux_Test_Sig/1 -> Converter control model/11(Aux_Test_Sig)
  Qinput_droop pu/1 -> inv_Scaling4/1
  PFAref/1 -> Converter control model/4(PFAref)
  WT_model/2(Pm) -> Scaling4/1
  WT_model/3(Cp) -> Cp/1
  WT_model/6(w_trip) -> w_trip/1
  WT_model/7(f_trip) -> f_trip/1
  Qref pu/1 -> inv_Scaling1/1
  WT_model/5(Pord) -> Converter control model/8(Pord)
  "Calculation of Power to network "/2(Qgen) -> Scaling2/1, Converter control model/6(Qgen)
  "Calculation of Power to network "/1(Pgen=Pelec) -> Scaling1/1, Divide2/1, WT_model/2(Pelec), Converter control model/5(Pelec)
  Generator_converter_model/1(Isorc) -> "Calculation of Power to network "/3(Isorc), Scaling3/1
  Complex to Magnitude-Angle/1 -> Converter control model/7(Vterm), "Calculation of Power to network "/1(absVterm)
  Vt pu/1 -> Generator_converter_model/3(V), "Calculation of Power to network "/2(Vterm), Complex to Magnitude-Angle/1
  Converter control model/2(Ipcmd) -> Generator_converter_model/2(Ipcmd)
  Converter control model/1(Eqcmd) -> Generator_converter_model/1(Eqcmd)
  "Calculation of Power to network "/3(Sgen) -> Abs/1
  Scaling1/1 -> Terminator5/1
  Scaling2/1 -> Terminator1/1

== system wtd_library_ver1/WTD Generator ver1 ==
  angle(elrad) : Inport
  Abs1 : Abs
  Abs_Eprim : Constant  Value=abs(E(co_node))
  Divide : Product  Inputs=*/
  Magnitude-Angle to Complex : MagnitudeAngleToComplex
  jXd : Constant  Value=jxd(co_node)
  Isorc pu : Outport
  wires:
  jXd/1 -> Divide/2
  Divide/1 -> Isorc pu/1
  Magnitude-Angle to Complex/1 -> Divide/1
  angle(elrad)/1 -> Magnitude-Angle to Complex/2
  Abs1/1 -> Magnitude-Angle to Complex/1
  Abs_Eprim/1 -> Abs1/1

== system wtd_library_ver1/WTD Hydro ver1 ==
  note: HYDRO 1
  "Pe pu " : Inport
  Add1 : Sum  Inputs=+-
  Add2 : Sum  Inputs=+-
  Gain : Gain  Gain=Sbasesys/Sbasem1
  Gain1 : Gain  Gain=Sbasem1/Sbasesys
  Gain2 : Gain  Gain=1/Sbasem1
  HYDRO turbine _HYGOV : Subsystem
  "Pm_init (MW) " : Constant  Value=Pm_init_vec(co_node)
  Rotor/Load2 : Subsystem
  delta_init (elrad)2 : Constant  Value=delta_init_vec(co_node)
  delta_w1 : Constant  Value=0
  Pm pu : Outport
  angle(elrad) : Outport  Port=2
  delta_w pu : Outport  Port=3
  wires:
  "Pm_init (MW) "/1 -> Gain2/1
  Gain2/1 -> Add2/2, Add1/2, HYDRO turbine _HYGOV/1(Pinit(pu mach.))
  delta_init (elrad)2/1 -> Rotor/Load2/3(angle(E)(elrad))
  Rotor/Load2/1(delta(elrad)) -> angle(elrad)/1
  Gain1/1 -> Pm pu/1
  "Pe pu "/1 -> Gain/1
  Gain/1 -> Add2/1
  delta_w1/1 -> Rotor/Load2/4(deltawro)
  Rotor/Load2/2(delta_w(pu)) -> HYDRO turbine _HYGOV/2(deltaw), delta_w pu/1
  Add1/1 -> Rotor/Load2/2(deltaPm(pu))
  Add2/1 -> Rotor/Load2/1("deltaPe(pu) ")
  HYDRO turbine _HYGOV/1(PMECH) -> Gain1/1, Add1/1
